simulink model "WPT_new"  (R2022b)
settings: Solver=VariableStepAuto  StartTime=0.0  StopTime=0.1  RelTol=1e-3
libraries: spsSeriesRLCBranchLib x26, spsDiodeLib x23, spsVoltageMeasurementLib x13, spsACVoltageSourceLib x5, spsMosfetLib x4, spsPWMGeneratorDCDCLib x4, spsMutualInductanceLib x3, spspowerguiLib x1
settings Model: Creator=SIDDHARTH  LastModifiedBy=SIDDHARTH

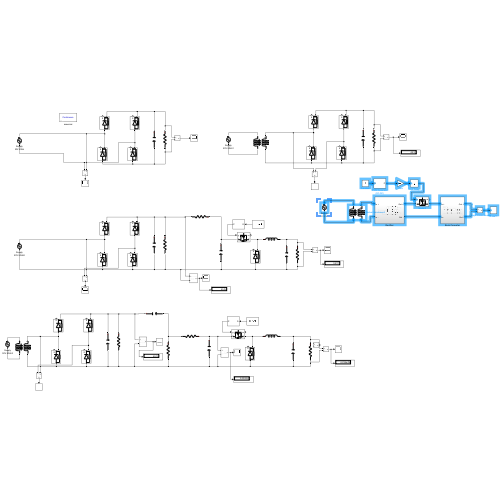
[thumbnail: Simulink's stored preview of the top-level diagram]
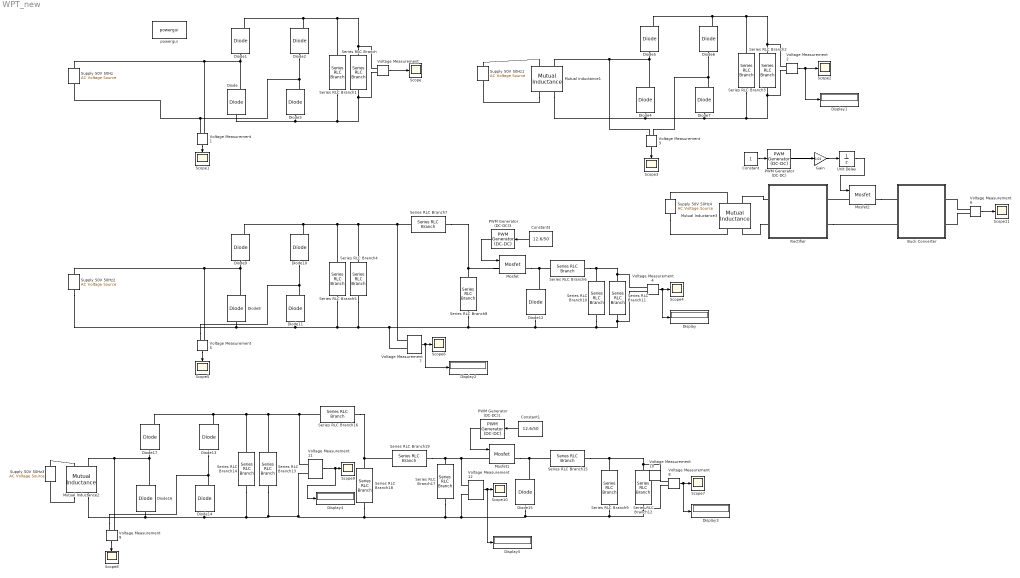
== system WPT_new ==
  Buck Converter : Subsystem
  Constant : Constant
  Constant1 : Constant  Value=12.6/50
  Constant3 : Constant  Value=12.6/50
  Diode{,2..4,6..8,10..16} (14 alike) : spsDiodeLib/Diode  Ron=0.001  Lon=0  Vf=0.7  IC=0  UseSnubber=0  Rs=500  Cs=250e-9  Measurements=on
  Diode{1,5,9,17} (4 alike) : spsDiodeLib/Diode  Ron=0.001  Lon=0  Vf=0.8  IC=0  UseSnubber=0  Rs=500  Cs=250e-9  Measurements=on
  Display{,1..5} (6 alike) : Display
  Gain : Gain  Gain=0.01
  Mosfet : spsMosfetLib/Mosfet  Ron=0.1  Lon=0  Rd=0.01  Vfd=0  IC=0  Rs=1e5  Cs=inf  Measurements=on
  Mosfet1 : spsMosfetLib/Mosfet  Ron=0.1  Lon=0  Rd=0.01  Vfd=0  IC=0  Rs=1e5  Cs=inf  Measurements=on
  Mosfet2 : spsMosfetLib/Mosfet  Ron=0.1  Lon=0  Rd=0.01  Vfd=0  IC=0  Rs=1e5  Cs=inf  Measurements=on
  Mutual Inductance1 : spsMutualInductanceLib/Mutual Inductance  LConnTagsString=a|b  RConnTagsString=A|B  TypeOfMutual=Two or three windings with equal mutual terms  NumberOfWindings=2  SelfImpedance1=[1.6054e-04 2.6286e-6]  SelfImpedance2=[1.6054e-04 2.6286e-6]  ThreeWindings=off  SelfImpedance3=[ 1.1 1.1e-03]  MutualImpedance=[1.5e-4 2.4264e-6]  InductanceMatrix="[1.0 0.9  0.9 ;  0.9 1.0  0.9;  0.9 0.9 1.0 ] * 1e-3"  ResistanceMatrix="[1.0 0.9  0.9 ;  0.9 1.0  0.9;  0.9 0.9 1.0 ]"  Measurements=None
      settings: LibrarySourceBlock=sps_lib/Passives/Mutual Inductance
  Mutual Inductance2 : spsMutualInductanceLib/Mutual Inductance  LConnTagsString=a|b  RConnTagsString=A|B  TypeOfMutual=Two or three windings with equal mutual terms  NumberOfWindings=2  SelfImpedance1=[1.1 15e-03]  SelfImpedance2=[ 1.1 15e-03]  ThreeWindings=off  SelfImpedance3=[ 1.1 1.1e-03]  MutualImpedance=[1.0 0.0138]  InductanceMatrix="[1.0 0.9  0.9 ;  0.9 1.0  0.9;  0.9 0.9 1.0 ] * 1e-3"  ResistanceMatrix="[1.0 0.9  0.9 ;  0.9 1.0  0.9;  0.9 0.9 1.0 ]"  Measurements=None
      settings: LibrarySourceBlock=sps_lib/Passives/Mutual Inductance
  Mutual Inductance3 : spsMutualInductanceLib/Mutual Inductance  LConnTagsString=a|b  RConnTagsString=A|B  TypeOfMutual=Two or three windings with equal mutual terms  NumberOfWindings=2  SelfImpedance1=[1.6054e-04 2.6286e-6]  SelfImpedance2=[1.6054e-04 2.6286e-6]  ThreeWindings=off  SelfImpedance3=[ 1.1 1.1e-03]  MutualImpedance=[1.5e-4 2.4264e-6]  InductanceMatrix="[1.0 0.9  0.9 ;  0.9 1.0  0.9;  0.9 0.9 1.0 ] * 1e-3"  ResistanceMatrix="[1.0 0.9  0.9 ;  0.9 1.0  0.9;  0.9 0.9 1.0 ]"  Measurements=None
      settings: LibrarySourceBlock=sps_lib/Passives/Mutual Inductance
  PWM Generator (DC-DC) : spsPWMGeneratorDCDCLib/PWM Generator (DC-DC)  Fsw=5000  Ts=0
  PWM Generator (DC-DC)1 : spsPWMGeneratorDCDCLib/PWM Generator (DC-DC)  Fsw=50000  Ts=0
  PWM Generator (DC-DC)3 : spsPWMGeneratorDCDCLib/PWM Generator (DC-DC)  Fsw=50000  Ts=0
  Rectifier : Subsystem
  Scope{,1..11} (12 alike) : Scope
  Series RLC Branch : spsSeriesRLCBranchLib/Series RLC Branch  LConnTagsString=__new0  RConnTagsString=__new0  BranchType=R  Resistance=100000  Inductance=1e-3  SetiL0=off  InitialCurrent=0  Capacitance=1e-6  Setx0=off  InitialVoltage=0  Measurements=None
  Series RLC Branch{1,3,5,8,14} (5 alike) : spsSeriesRLCBranchLib/Series RLC Branch  LConnTagsString=__new0  RConnTagsString=__new0  BranchType=C  Resistance=1  Inductance=1e-3  SetiL0=off  InitialCurrent=0  Capacitance=100e-6  Setx0=off  InitialVoltage=0  Measurements=Branch voltage
  Series RLC Branch10 : spsSeriesRLCBranchLib/Series RLC Branch  LConnTagsString=__new0  RConnTagsString=__new0  BranchType=C  Resistance=1  Inductance=1e-3  SetiL0=off  InitialCurrent=0  Capacitance=220e-6  Setx0=off  InitialVoltage=0  Measurements=None
  Series RLC Branch11 : spsSeriesRLCBranchLib/Series RLC Branch  LConnTagsString=__new0  RConnTagsString=__new0  BranchType=R  Resistance=1  Inductance=1e-3  SetiL0=off  InitialCurrent=0  Capacitance=1e-6  Setx0=off  InitialVoltage=0  Measurements=None
  Series RLC Branch12 : spsSeriesRLCBranchLib/Series RLC Branch  LConnTagsString=__new0  RConnTagsString=__new0  BranchType=R  Resistance=1  Inductance=1e-3  SetiL0=off  InitialCurrent=0  Capacitance=1e-6  Setx0=off  InitialVoltage=0  Measurements=None
  Series RLC Branch13 : spsSeriesRLCBranchLib/Series RLC Branch  LConnTagsString=__new0  RConnTagsString=__new0  BranchType=R  Resistance=1000000  Inductance=1e-3  SetiL0=off  InitialCurrent=0  Capacitance=1e-6  Setx0=off  InitialVoltage=0  Measurements=None
  Series RLC Branch15 : spsSeriesRLCBranchLib/Series RLC Branch  LConnTagsString=__new0  RConnTagsString=__new0  BranchType=L  Resistance=1  Inductance=33e-6  SetiL0=off  InitialCurrent=0  Capacitance=1e-6  Setx0=off  InitialVoltage=0  Measurements=None
  Series RLC Branch16 : spsSeriesRLCBranchLib/Series RLC Branch  LConnTagsString=__new0  RConnTagsString=__new0  BranchType=C  Resistance=1  Inductance=1e-3  SetiL0=off  InitialCurrent=0  Capacitance=100e-9  Setx0=off  InitialVoltage=0  Measurements=Branch voltage
  Series RLC Branch17 : spsSeriesRLCBranchLib/Series RLC Branch  LConnTagsString=__new0  RConnTagsString=__new0  BranchType=C  Resistance=1  Inductance=1e-3  SetiL0=off  InitialCurrent=0  Capacitance=100e-9  Setx0=off  InitialVoltage=0  Measurements=Branch voltage
  Series RLC Branch18 : spsSeriesRLCBranchLib/Series RLC Branch  LConnTagsString=__new0  RConnTagsString=__new0  BranchType=R  Resistance=127.32e3  Inductance=1e-3  SetiL0=off  InitialCurrent=0  Capacitance=1e-6  Setx0=off  InitialVoltage=0  Measurements=None
  Series RLC Branch19 : spsSeriesRLCBranchLib/Series RLC Branch  LConnTagsString=__new0  RConnTagsString=__new0  BranchType=R  Resistance=123.98e3  Inductance=1e-3  SetiL0=off  InitialCurrent=0  Capacitance=1e-6  Setx0=off  InitialVoltage=0  Measurements=None
  Series RLC Branch2 : spsSeriesRLCBranchLib/Series RLC Branch  LConnTagsString=__new0  RConnTagsString=__new0  BranchType=R  Resistance=100000  Inductance=1e-3  SetiL0=off  InitialCurrent=0  Capacitance=1e-6  Setx0=off  InitialVoltage=0  Measurements=None
  Series RLC Branch4 : spsSeriesRLCBranchLib/Series RLC Branch  LConnTagsString=__new0  RConnTagsString=__new0  BranchType=R  Resistance=1000000  Inductance=1e-3  SetiL0=off  InitialCurrent=0  Capacitance=1e-6  Setx0=off  InitialVoltage=0  Measurements=None
  Series RLC Branch6 : spsSeriesRLCBranchLib/Series RLC Branch  LConnTagsString=__new0  RConnTagsString=__new0  BranchType=L  Resistance=1  Inductance=33e-6  SetiL0=off  InitialCurrent=0  Capacitance=1e-6  Setx0=off  InitialVoltage=0  Measurements=None
  Series RLC Branch7 : spsSeriesRLCBranchLib/Series RLC Branch  LConnTagsString=__new0  RConnTagsString=__new0  BranchType=R  Resistance=318.3  Inductance=1e-3  SetiL0=off  InitialCurrent=0  Capacitance=1e-6  Setx0=off  InitialVoltage=0  Measurements=None
  Series RLC Branch9 : spsSeriesRLCBranchLib/Series RLC Branch  LConnTagsString=__new0  RConnTagsString=__new0  BranchType=C  Resistance=1  Inductance=1e-3  SetiL0=off  InitialCurrent=0  Capacitance=220e-6  Setx0=off  InitialVoltage=0  Measurements=None
  Supply 50V 50Hz{,1..4} (5 alike) : spsACVoltageSourceLib/AC Voltage Source  Amplitude=50  Phase=0  Frequency=50  SampleTime=0  Measurements=None  BusType=swing  Pref=10e3  Qref=0  Qmin=-inf  Qmax=+inf
  Unit Delay : UnitDelay  SampleTime=-1  HasFrameUpgradeWarning=on
  Voltage Measurement{,1..12} (13 alike) : spsVoltageMeasurementLib/Voltage Measurement  PhasorSimulation=off  OutputType=Complex  PSBequivalent=0
  powergui : spspowerguiLib/powergui  Priority=1  SimulationMode=Continuous  SampleTime=50e-6  frequency=60  Iterations=50  frequencyindice=0  Pbase=100e6  ErrMax=1e-4  UnitsV=kV  UnitsW=MW  buscounter=0  FunctionMessages=off  echomessages=off  EnableUseOfTLC=off  CurrentSourceSwitches=off  DisableSnubberDevices=off  DisableRonSwitches=off  DisableVfSwitches=off  DisplayEquations=off  AutomaticDiscreteSolvers=off  SolverType=Tustin/Backward Euler (TBE)  Interpol=off  ExternalGateDelay=off  methode=off  Ts=100  x0status=blocks  SPID=on  SwTol=0  HookPort=off  NonlinearTolerance=1e-4  nMaxIteration=100  ContinueOnMaxIteration=off  RestoreLinks=warning  ResistiveCurrentMeasurement=off  Frange=[0:2:500]  Ylog=off  Xlog=on  ShowGrid=off  save=off  variable=ZData  structure=0  ZoomFFT=off  StartTime=0.0  cycles=1  DisplayStyle=1  fundamental=60  FreqAxis=off  MaxFrequency=1000  frequencyindicesteady=1  RmsSteady=1  display=off
  wires:
  Voltage Measurement1/1 -> Scope1/1
  Voltage Measurement/1 -> Scope/1
  Voltage Measurement2/1 -> Display1/1, Scope2/1
  Voltage Measurement3/1 -> Scope3/1
  Voltage Measurement5/1 -> Scope5/1
  Constant3/1 -> PWM Generator (DC-DC)3/1
  PWM Generator (DC-DC)3/1 -> Mosfet/1
  Voltage Measurement4/1 -> Display/1, Scope4/1
  Voltage Measurement7/1 -> Display2/1, Scope6/1
  Voltage Measurement9/1 -> Scope8/1
  Voltage Measurement11/1 -> Display4/1, Scope9/1
  Voltage Measurement8/1 -> Display3/1, Scope7/1
  Constant1/1 -> PWM Generator (DC-DC)1/1
  PWM Generator (DC-DC)1/1 -> Mosfet1/1
  Voltage Measurement12/1 -> Display5/1, Scope10/1
  Voltage Measurement6/1 -> Scope11/1
  Constant/1 -> PWM Generator (DC-DC)/1
  PWM Generator (DC-DC)/1 -> Gain/1
  Unit Delay/1 -> Mosfet2/1
  Gain/1 -> Unit Delay/1
  connections:
  Supply 50V 50Hz/LConn1 -- Diode3/RConn1 -- Diode2/LConn1 -- Voltage Measurement1/LConn2
  Series RLC Branch/LConn1 -- Voltage Measurement/LConn1 -- Series RLC Branch1/LConn1 -- Diode1/RConn1 -- Diode2/RConn1
  Diode3/LConn1 -- Diode/LConn1 -- Series RLC Branch/RConn1 -- Voltage Measurement/LConn2 -- Series RLC Branch1/RConn1
  Diode1/LConn1 -- Diode/RConn1 -- Supply 50V 50Hz/RConn1 -- Voltage Measurement1/LConn1
  Diode7/LConn1 -- Mutual Inductance1/RConn2 -- Diode4/LConn1 -- Series RLC Branch3/RConn1 -- Series RLC Branch2/RConn1 -- Voltage Measurement2/LConn2
  Diode5/LConn1 -- Mutual Inductance1/LConn2 -- Voltage Measurement3/LConn1 -- Diode4/RConn1
  Diode6/RConn1 -- Diode5/RConn1 -- Series RLC Branch3/LConn1 -- Voltage Measurement2/LConn1 -- Series RLC Branch2/LConn1
  Voltage Measurement3/LConn2 -- Diode7/RConn1 -- Diode6/LConn1
  Mutual Inductance1/LConn1 -- Supply 50V 50Hz1/RConn1
  Mutual Inductance1/RConn1 -- Supply 50V 50Hz1/LConn1
  Voltage Measurement5/LConn2 -- Diode11/RConn1 -- Diode10/LConn1
  Diode10/RConn1 -- Diode9/RConn1 -- Series RLC Branch5/LConn1 -- Voltage Measurement7/LConn1 -- Series RLC Branch7/RConn1 -- Series RLC Branch4/LConn1
  Diode12/LConn1 -- Series RLC Branch8/RConn1 -- Series RLC Branch5/RConn1 -- Supply 50V 50Hz2/LConn1 -- Diode8/LConn1 -- Diode11/LConn1 -- Series RLC Branch4/RConn1 -- Voltage Measurement7/LConn2 -- Voltage Measurement4/LConn2 -- Series RLC Branch11/RConn1 -- Series RLC Branch10/RConn1
  Diode9/LConn1 -- Supply 50V 50Hz2/RConn1 -- Voltage Measurement5/LConn1 -- Diode8/RConn1
  Series RLC Branch6/RConn1 -- Voltage Measurement4/LConn1 -- Series RLC Branch11/LConn1 -- Series RLC Branch10/LConn1
  Mosfet/RConn1 -- Diode12/RConn1 -- Series RLC Branch6/LConn1
  Series RLC Branch7/LConn1 -- Mosfet/LConn1 -- Series RLC Branch8/LConn1
  Diode17/LConn1 -- Mutual Inductance2/LConn2 -- Voltage Measurement9/LConn1 -- Diode16/RConn1
  Series RLC Branch14/RConn1 -- Voltage Measurement12/LConn2 -- Diode15/LConn1 -- Series RLC Branch9/RConn1 -- Voltage Measurement8/LConn2 -- Series RLC Branch12/RConn1 -- Series RLC Branch17/RConn1 -- Series RLC Branch18/RConn1 -- Voltage Measurement11/LConn2 -- Series RLC Branch13/RConn1 -- Mutual Inductance2/RConn2 -- Diode16/LConn1 -- Diode14/LConn1
  Voltage Measurement9/LConn2 -- Diode14/RConn1 -- Diode13/LConn1
  Series RLC Branch12/LConn1 -- Voltage Measurement8/LConn1 -- Series RLC Branch9/LConn1 -- Series RLC Branch15/RConn1
  Diode13/RConn1 -- Diode17/RConn1 -- Series RLC Branch14/LConn1 -- Series RLC Branch16/LConn1 -- Voltage Measurement11/LConn1 -- Series RLC Branch13/LConn1
  Mosfet1/RConn1 -- Diode15/RConn1 -- Series RLC Branch15/LConn1
  Series RLC Branch17/LConn1 -- Voltage Measurement12/LConn1 -- Mosfet1/LConn1 -- Series RLC Branch19/LConn1
  Series RLC Branch16/RConn1 -- Series RLC Branch19/RConn1 -- Series RLC Branch18/LConn1
  Supply 50V 50Hz3/RConn1 -- Mutual Inductance2/LConn1
  Mutual Inductance2/RConn1 -- Supply 50V 50Hz3/LConn1
  Supply 50V 50Hz4/LConn1 -- Mutual Inductance3/RConn1
  Mutual Inductance3/LConn1 -- Supply 50V 50Hz4/RConn1
  Mutual Inductance3/LConn2 -- Rectifier/LConn1
  Rectifier/LConn2 -- Mutual Inductance3/RConn2
  Rectifier/RConn2 -- Buck Converter/LConn2
  Voltage Measurement6/LConn1 -- Buck Converter/RConn1
  Voltage Measurement6/LConn2 -- Buck Converter/RConn2
  Mosfet2/LConn1 -- Rectifier/RConn1
  Mosfet2/RConn1 -- Buck Converter/LConn1

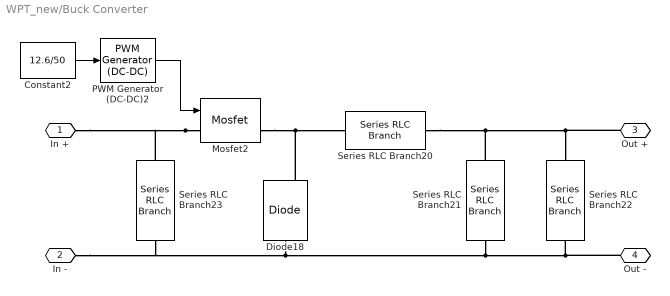
== system WPT_new/Buck Converter ==
  Constant2 : Constant  Value=12.6/50
  Diode18 : spsDiodeLib/Diode  Ron=0.001  Lon=0  Vf=0  IC=0  UseSnubber=0  Rs=500  Cs=250e-9  Measurements=on
  Mosfet2 : spsMosfetLib/Mosfet  Ron=0.1  Lon=0  Rd=0.01  Vfd=0  IC=0  Rs=1e5  Cs=inf  Measurements=on
  PWM Generator (DC-DC)2 : spsPWMGeneratorDCDCLib/PWM Generator (DC-DC)  Fsw=50000  Ts=0
  Series RLC Branch20 : spsSeriesRLCBranchLib/Series RLC Branch  LConnTagsString=__new0  RConnTagsString=__new0  BranchType=L  Resistance=1  Inductance=33e-6  SetiL0=off  InitialCurrent=0  Capacitance=1e-6  Setx0=off  InitialVoltage=0  Measurements=None
  Series RLC Branch21 : spsSeriesRLCBranchLib/Series RLC Branch  LConnTagsString=__new0  RConnTagsString=__new0  BranchType=C  Resistance=1  Inductance=1e-3  SetiL0=off  InitialCurrent=0  Capacitance=220e-6  Setx0=off  InitialVoltage=0  Measurements=None
  Series RLC Branch22 : spsSeriesRLCBranchLib/Series RLC Branch  LConnTagsString=__new0  RConnTagsString=__new0  BranchType=R  Resistance=1  Inductance=1e-3  SetiL0=off  InitialCurrent=0  Capacitance=1e-6  Setx0=off  InitialVoltage=0  Measurements=None
  Series RLC Branch23 : spsSeriesRLCBranchLib/Series RLC Branch  LConnTagsString=__new0  RConnTagsString=__new0  BranchType=RC  Resistance=0.0001  Inductance=1e-3  SetiL0=off  InitialCurrent=0  Capacitance=100e-6  Setx0=off  InitialVoltage=0  Measurements=None
  In + : PMIOPort  Side=Left
  In - : PMIOPort  Port=2  Side=Left
  Out + : PMIOPort  Port=3  Side=Right
  Out - : PMIOPort  Port=4  Side=Right
  wires:
  Constant2/1 -> PWM Generator (DC-DC)2/1
  PWM Generator (DC-DC)2/1 -> Mosfet2/1
  connections:
  Mosfet2/LConn1 -- In +/RConn1 -- Series RLC Branch23/LConn1
  Diode18/LConn1 -- In -/RConn1 -- Series RLC Branch23/RConn1 -- Series RLC Branch21/RConn1 -- Out -/RConn1 -- Series RLC Branch22/RConn1
  Series RLC Branch20/RConn1 -- Series RLC Branch21/LConn1 -- Out +/RConn1 -- Series RLC Branch22/LConn1
  Mosfet2/RConn1 -- Diode18/RConn1 -- Series RLC Branch20/LConn1

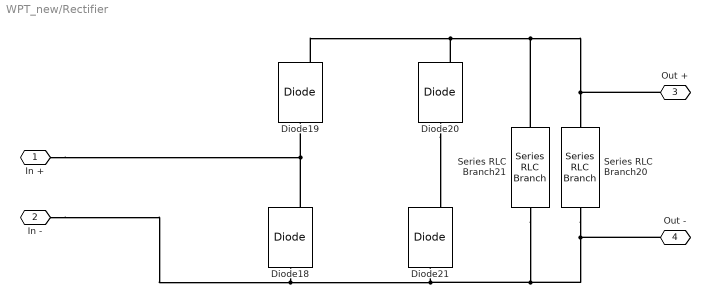
== system WPT_new/Rectifier ==
  Diode18 : spsDiodeLib/Diode  Ron=0.001  Lon=0  Vf=0.7  IC=0  UseSnubber=0  Rs=500  Cs=250e-9  Measurements=on
  Diode19 : spsDiodeLib/Diode  Ron=0.001  Lon=0  Vf=0.8  IC=0  UseSnubber=0  Rs=500  Cs=250e-9  Measurements=on
  Diode20 : spsDiodeLib/Diode  Ron=0.001  Lon=0  Vf=0.7  IC=0  UseSnubber=0  Rs=500  Cs=250e-9  Measurements=on
  Diode21 : spsDiodeLib/Diode  Ron=0.001  Lon=0  Vf=0.7  IC=0  UseSnubber=0  Rs=500  Cs=250e-9  Measurements=on
  Series RLC Branch20 : spsSeriesRLCBranchLib/Series RLC Branch  LConnTagsString=__new0  RConnTagsString=__new0  BranchType=R  Resistance=100000  Inductance=1e-3  SetiL0=off  InitialCurrent=0  Capacitance=1e-6  Setx0=off  InitialVoltage=0  Measurements=None
  Series RLC Branch21 : spsSeriesRLCBranchLib/Series RLC Branch  LConnTagsString=__new0  RConnTagsString=__new0  BranchType=C  Resistance=1  Inductance=1e-3  SetiL0=off  InitialCurrent=0  Capacitance=100e-6  Setx0=off  InitialVoltage=0  Measurements=Branch voltage
  In + : PMIOPort  Side=Left
  In - : PMIOPort  Port=2  Side=Left
  Out + : PMIOPort  Port=3  Side=Right
  Out - : PMIOPort  Port=4  Side=Right
  connections:
  Diode20/RConn1 -- Diode19/RConn1 -- Series RLC Branch21/LConn1 -- Out +/RConn1 -- Series RLC Branch20/LConn1
  Series RLC Branch20/RConn1 -- Out -/RConn1 -- Series RLC Branch21/RConn1 -- In -/RConn1 -- Diode18/LConn1 -- Diode21/LConn1
  Diode18/RConn1 -- Diode19/LConn1 -- In +/RConn1
  Diode20/LConn1 -- Diode21/RConn1
